simulink library "wtd_library_ver1"  (R2014b)
settings: Solver=ode45  StartTime=0.0  StopTime=10.0  RelTol=1e-3
undefined symbols (not defined in the file or in its folder): clearaugYMatrix, complexPower, dwo, faultaugYMatrix, genTranReactance, invclearaugYMatrix, invfaultaugYMatrix, invsystemaugYMatrix, j, nodeVoltage, noGridNodes, pffault_set_global, s3cc, tho
undefined symbols (not defined in the file): baseSystemPower, internalGenVoltage, pitchAngleVec, systemFrequency, turbSpeedVec, windturbKaParam, windturbKbParam, WTD_Y12, WTD_Y12_2
libraries: simulink x18
(part 3 of 3)

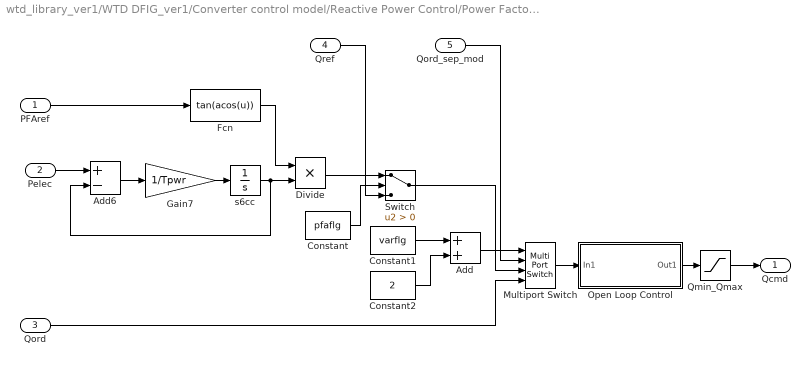
== system wtd_library_ver1/WTD DFIG_ver1/Converter control model/Reactive Power Control/Power Factor Regulator ==
  PFAref : Inport
  Pelec : Inport  Port=2
  Qord : Inport  Port=3
  Qref : Inport  Port=4
  Qord_sep_mod : Inport  Port=5
  Add : Sum
  Add6 : Sum  Inputs=+-
  Constant : Constant  Value=pfaflg
  Constant1 : Constant  Value=varflg
  Constant2 : Constant  Value=2
  Divide : Product  Inputs=**
  Fcn : Fcn  Expr=tan(acos(u))
  Gain7 : Gain  Gain=1/Tpwr
  Multiport Switch : MultiPortSwitch
  Open Loop Control : Subsystem
  Qmin_Qmax : Saturate  UpperLimit=Qmax  LowerLimit=Qmin
  Switch : Switch  Criteria=u2 > Threshold
  s6cc : Integrator  InitialCondition=s6cc
  Qcmd : Outport
  wires:
  Pelec/1 -> Add6/1
  s6cc/1 -> Divide/2, Add6/2
  Add6/1 -> Gain7/1
  Gain7/1 -> s6cc/1
  Qmin_Qmax/1 -> Qcmd/1
  Open Loop Control/1(Out1) -> Qmin_Qmax/1
  Multiport Switch/1 -> Open Loop Control/1(In1)
  Qord/1 -> Multiport Switch/4
  Switch/1 -> Multiport Switch/3
  Qord_sep_mod/1 -> Multiport Switch/2
  Add/1 -> Multiport Switch/1
  Constant2/1 -> Add/2
  Constant1/1 -> Add/1
  Qref/1 -> Switch/3
  Constant/1 -> Switch/2
  Divide/1 -> Switch/1
  Fcn/1 -> Divide/1
  PFAref/1 -> Fcn/1

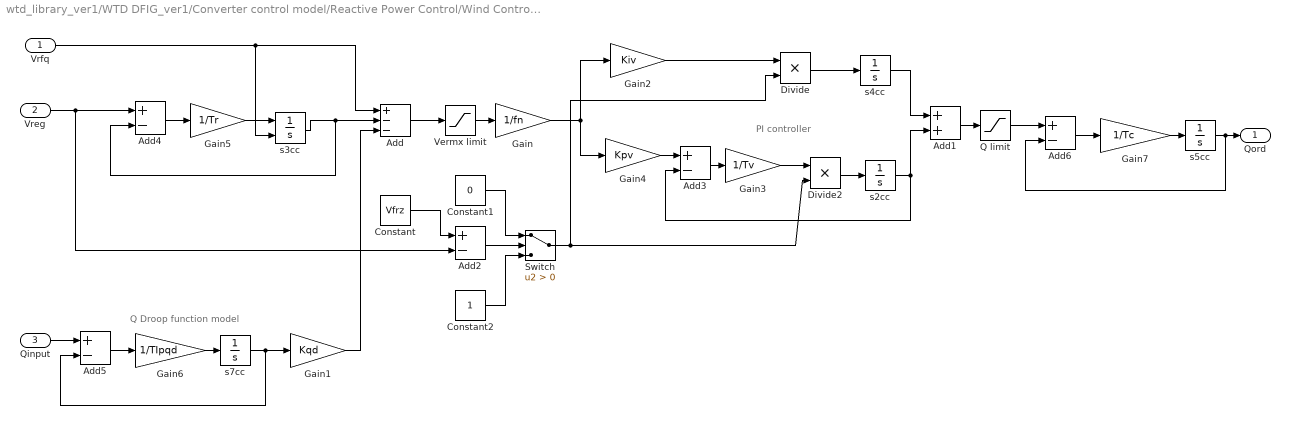
== system wtd_library_ver1/WTD DFIG_ver1/Converter control model/Reactive Power Control/Wind Control Emulator ==
  note: PI controller
  note: Q Droop function model
  Vrfq : Inport
  Vreg : Inport  Port=2
  Qinput : Inport  Port=3
  Add : Sum  Inputs=+--
  Add1 : Sum
  Add{2..6} (5 alike) : Sum  Inputs=+-
  Constant : Constant  Value=Vfrz
  Constant1 : Constant  Value=0
  Constant2 : Constant
  Divide : Product  Inputs=**
  Divide2 : Product  Inputs=**
  Gain : Gain  Gain=1/fn
  Gain1 : Gain  Gain=Kqd
  Gain2 : Gain  Gain=Kiv
  Gain3 : Gain  Gain=1/Tv
  Gain4 : Gain  Gain=Kpv
  Gain5 : Gain  Gain=1/Tr
  Gain6 : Gain  Gain=1/TIpqd
  Gain7 : Gain  Gain=1/Tc
  Q limit : Saturate  UpperLimit=Qmax  LowerLimit=Qmin
  Switch : Switch  Criteria=u2 > Threshold
  Vermx limit : Saturate  UpperLimit=Vermx  LowerLimit=Vermn
  s2cc : Integrator  InitialCondition=s2cc
  s3cc : Integrator  InitialConditionSource=external  InitialCondition=s3cc
  s4cc : Integrator  InitialCondition=s4cc
  s5cc : Integrator  InitialCondition=s5cc
  s7cc : Integrator  InitialCondition=s7cc
  Qord : Outport
  wires:
  Q limit/1 -> Add6/1
  s5cc/1 -> Qord/1, Add6/2
  Add6/1 -> Gain7/1
  Gain7/1 -> s5cc/1
  Qinput/1 -> Add5/1
  s7cc/1 -> Gain1/1, Add5/2
  Add5/1 -> Gain6/1
  Gain6/1 -> s7cc/1
  s3cc/1 -> Add/2, Add4/2
  Add4/1 -> Gain5/1
  Gain5/1 -> s3cc/1
  Divide/1 -> s4cc/1
  Gain2/1 -> Divide/1
  Constant2/1 -> Switch/3
  Switch/1 -> Divide2/2, Divide/2
  Gain4/1 -> Add3/1
  Add3/1 -> Gain3/1
  s2cc/1 -> Add1/2, Add3/2
  Divide2/1 -> s2cc/1
  Gain3/1 -> Divide2/1
  Constant1/1 -> Switch/1
  Constant/1 -> Add2/1
  Add2/1 -> Switch/2
  Add1/1 -> Q limit/1
  s4cc/1 -> Add1/1
  Gain/1 -> Gain2/1, Gain4/1
  Gain1/1 -> Add/3
  Vermx limit/1 -> Gain/1
  Add/1 -> Vermx limit/1
  Vreg/1 -> Add4/1, Add2/2
  Vrfq/1 -> Add/1, s3cc/2

== system wtd_library_ver1/WTD DFIG_ver1/WT_model/Active Power Control Emulator/Subsystem ==
  pavf : Inport
  fbu : Inport  Port=2
  0 : Constant  Value=0
  1 : Constant
  Add : Sum  Inputs=+-
  Divide : Product  Inputs=**
  Fd : Constant  Value=Fd
  Lookup Table1 : Lookup  InputValues=[0.95 Fa Fb Fc Fd]  Table=[Pa Pa Pbc Pbc Pd]
  Switch : Switch  Criteria=u2 > Threshold
  Timer 1 s : Subsystem
  pset : Outport
  f_trip : Outport  Port=2
  wires:
  1/1 -> Switch/1
  0/1 -> Switch/3
  Add/1 -> Switch/2
  Fd/1 -> Add/2
  Switch/1 -> Timer 1 s/1(enable)
  Divide/1 -> pset/1
  Lookup Table1/1 -> Divide/2
  pavf/1 -> Divide/1
  fbu/1 -> Lookup Table1/1, Add/1
  Timer 1 s/1(f_trip) -> f_trip/1

== system wtd_library_ver1/WTD DFIG_ver1/WT_model/Active Power Control Emulator/Wind power model1 ==
  vw : Inport
  Cpmax : Constant  Value=0.5173
  Divide1 : Product  Inputs=***
  Fcn : Fcn  Expr=u^3
  Ka : Constant  Value=Ka(co_node)
  Pmech : Outport
  wires:
  Cpmax/1 -> Divide1/2
  Divide1/1 -> Pmech/1  "Pmech"
  Fcn/1 -> Divide1/1
  Ka/1 -> Divide1/3
  vw/1 -> Fcn/1

== system wtd_library_ver1/WTD DFIG_ver1/WT_model/Pitch compensator/Saturation ==
  z : Inport
  ymax : Inport  Port=2
  ymin : Inport  Port=3
  y : Inport  Port=4
  Add1 : Sum
  Add2 : Sum  Inputs=-+
  Add3 : Sum  Inputs=+-
  Add4 : Sum
  Compare To Zero : simulink/Logic and Bit Operations/Compare To Zero  relop=<  OutDataTypeStr=uint8
  Compare To Zero1 : simulink/Logic and Bit Operations/Compare To Zero  relop=<  OutDataTypeStr=uint8
  Compare To Zero{2..5} (4 alike) : simulink/Logic and Bit Operations/Compare To Zero  relop=>  OutDataTypeStr=uint8
  Product : Product  RndMeth=Zero
  ysw : Outport
  wires:
  Product/1 -> ysw/1
  Compare To Zero5/1 -> Product/2
  Compare To Zero2/1 -> Product/1
  Add4/1 -> Compare To Zero5/1
  Compare To Zero3/1 -> Add4/2
  Compare To Zero4/1 -> Add4/1
  Add3/1 -> Compare To Zero3/1
  ymin/1 -> Add3/2
  Add1/1 -> Compare To Zero2/1
  Compare To Zero/1 -> Add1/2
  Compare To Zero1/1 -> Add1/1
  z/1 -> Compare To Zero4/1, Compare To Zero/1
  Add2/1 -> Compare To Zero1/1
  ymax/1 -> Add2/1
  y/1 -> Add3/1, Add2/2

== system wtd_library_ver1/WTD DFIG_ver1/WT_model/Pitch controller/Saturation ==
  z : Inport
  ymax : Inport  Port=2
  ymin : Inport  Port=3
  y : Inport  Port=4
  Add1 : Sum
  Add2 : Sum  Inputs=-+
  Add3 : Sum  Inputs=+-
  Add4 : Sum
  Compare To Zero : simulink/Logic and Bit Operations/Compare To Zero  relop=<  OutDataTypeStr=uint8
  Compare To Zero1 : simulink/Logic and Bit Operations/Compare To Zero  relop=<  OutDataTypeStr=uint8
  Compare To Zero{2..5} (4 alike) : simulink/Logic and Bit Operations/Compare To Zero  relop=>  OutDataTypeStr=uint8
  Product : Product  RndMeth=Zero
  ysw : Outport
  wires:
  Product/1 -> ysw/1
  Compare To Zero5/1 -> Product/2
  Compare To Zero2/1 -> Product/1
  Add4/1 -> Compare To Zero5/1
  Compare To Zero3/1 -> Add4/2
  Compare To Zero4/1 -> Add4/1
  Add3/1 -> Compare To Zero3/1
  ymin/1 -> Add3/2
  Add1/1 -> Compare To Zero2/1
  Compare To Zero/1 -> Add1/2
  Compare To Zero1/1 -> Add1/1
  z/1 -> Compare To Zero4/1, Compare To Zero/1
  Add2/1 -> Compare To Zero1/1
  ymax/1 -> Add2/1
  y/1 -> Add3/1, Add2/2

== system wtd_library_ver1/WTD DFIG_ver1/WT_model/Torque controller/Saturation ==
  z : Inport
  ymax : Inport  Port=2
  ymin : Inport  Port=3
  y : Inport  Port=4
  Add1 : Sum
  Add2 : Sum  Inputs=-+
  Add3 : Sum  Inputs=+-
  Add4 : Sum
  Compare To Zero : simulink/Logic and Bit Operations/Compare To Zero  relop=<  OutDataTypeStr=uint8
  Compare To Zero1 : simulink/Logic and Bit Operations/Compare To Zero  relop=<  OutDataTypeStr=uint8
  Compare To Zero{2..5} (4 alike) : simulink/Logic and Bit Operations/Compare To Zero  relop=>  OutDataTypeStr=uint8
  Product : Product  RndMeth=Zero
  ysw : Outport
  wires:
  Product/1 -> ysw/1
  Compare To Zero5/1 -> Product/2
  Compare To Zero2/1 -> Product/1
  Add4/1 -> Compare To Zero5/1
  Compare To Zero3/1 -> Add4/2
  Compare To Zero4/1 -> Add4/1
  Add3/1 -> Compare To Zero3/1
  ymin/1 -> Add3/2
  Add1/1 -> Compare To Zero2/1
  Compare To Zero/1 -> Add1/2
  Compare To Zero1/1 -> Add1/1
  z/1 -> Compare To Zero4/1, Compare To Zero/1
  Add2/1 -> Compare To Zero1/1
  ymax/1 -> Add2/1
  y/1 -> Add3/1, Add2/2

== system wtd_library_ver1/WTD DFIG_ver1/WT_model/Wind power model/Cp & lambda ==
  theta : Inport
  vw : Inport  Port=2
  w : Inport  Port=3
  Product : Product  Inputs=3  Multiplication=Matrix(*)  RndMeth=Zero
  Vektor lambda : Subsystem
  Vektor theta : Subsystem
  cp_koeficijenti : Constant  Value=alpha
  Cp : Outport
  lambda : Outport  Port=2
  wires:
  Vektor lambda/1(lambda) -> lambda/1
  Product/1 -> Cp/1
  w/1 -> Vektor lambda/2(w)
  vw/1 -> Vektor lambda/1(vw)
  theta/1 -> Vektor theta/1(theta)
  cp_koeficijenti/1 -> Product/2
  Vektor lambda/2(lambda_na_j) -> Product/3
  Vektor theta/1(theta_na_i) -> Product/1

== system wtd_library_ver1/WTD DFIG_ver1/Converter control model/Reactive Power Control/Power Factor Regulator/Open Loop Control ==
  In1 : Inport
  Out1 : Outport
  wires:
  In1/1 -> Out1/1

== system wtd_library_ver1/WTD DFIG_ver1/WT_model/Active Power Control Emulator/Subsystem/Timer 1 s ==
  enable : Inport
  Add : Sum  Inputs=-+
  Constant2 : Constant
  Constant3 : Constant  Value=0
  Enabled Subsystem : Subsystem  TreatAsAtomicUnit=on
  Enabled Subsystem1 : Subsystem  TreatAsAtomicUnit=on
  Hit Crossing : HitCross  HitCrossingDirection=rising
  Switch : Switch  Threshold=1
  f_trip : Outport
  wires:
  Hit Crossing/1 -> Enabled Subsystem/Enable
  Enabled Subsystem/1(timer) -> Add/1
  Enabled Subsystem1/1(timer) -> Add/2
  Switch/1 -> f_trip/1
  Add/1 -> Switch/2
  Constant2/1 -> Switch/1
  Constant3/1 -> Switch/3
  enable/1 -> Hit Crossing/1, Enabled Subsystem1/Enable

== system wtd_library_ver1/WTD DFIG_ver1/WT_model/Wind power model/Cp & lambda/Vektor lambda ==
  vw : Inport
  w : Inport  Port=2
  Constant1 : Constant
  Divide1 : Product  Inputs=/*
  Divide2 : Product  Inputs=**
  Divide3 : Product  Inputs=**
  Divide4 : Product  Inputs=**
  Gain : Gain  Gain=Kb(co_node)
  Reshape : Reshape  OutputDimensionality=Customize  OutputDimensions=[5,1]
  Vector Concatenate : Concatenate  NumInputs=5
  lambda : Outport
  lambda_na_j : Outport  Port=2
  wires:
  Reshape/1 -> lambda_na_j/1
  Vector Concatenate/1 -> Reshape/1
  vw/1 -> Divide1/1
  w/1 -> Divide1/2
  Divide4/1 -> Vector Concatenate/5
  Divide3/1 -> Divide4/1, Vector Concatenate/4
  Divide2/1 -> Divide3/1, Vector Concatenate/3
  Gain/1 -> lambda/1, Divide4/2, Divide3/2, Divide2/2, Divide2/1, Vector Concatenate/2
  Constant1/1 -> Vector Concatenate/1
  Divide1/1 -> Gain/1

== system wtd_library_ver1/WTD DFIG_ver1/WT_model/Wind power model/Cp & lambda/Vektor theta ==
  theta : Inport
  Constant1 : Constant
  Divide2 : Product  Inputs=**
  Divide3 : Product  Inputs=**
  Divide4 : Product  Inputs=**
  Reshape : Reshape  OutputDimensionality=Customize  OutputDimensions=[1,5]
  Vector Concatenate : Concatenate  NumInputs=5
  theta_na_i : Outport
  wires:
  Reshape/1 -> theta_na_i/1
  Vector Concatenate/1 -> Reshape/1
  Constant1/1 -> Vector Concatenate/1
  Divide2/1 -> Vector Concatenate/3, Divide3/1
  Divide3/1 -> Vector Concatenate/4, Divide4/1
  Divide4/1 -> Vector Concatenate/5
  theta/1 -> Vector Concatenate/2, Divide2/1, Divide2/2, Divide3/2, Divide4/2

== system wtd_library_ver1/WTD DFIG_ver1/WT_model/Active Power Control Emulator/Subsystem/Timer 1 s/Enabled Subsystem ==
  Enable : EnablePort
  Constant : Constant
  Enabled Subsystem : Subsystem  TreatAsAtomicUnit=on
  timer : Outport
  wires:
  Enabled Subsystem/1(Out1) -> timer/1
  Constant/1 -> Enabled Subsystem/Enable

== system wtd_library_ver1/WTD DFIG_ver1/WT_model/Active Power Control Emulator/Subsystem/Timer 1 s/Enabled Subsystem1 ==
  Enable : EnablePort
  Clock : Clock
  timer : Outport
  wires:
  Clock/1 -> timer/1

== system wtd_library_ver1/WTD DFIG_ver1/WT_model/Active Power Control Emulator/Subsystem/Timer 1 s/Enabled Subsystem/Enabled Subsystem ==
  Enable : EnablePort
  Clock : Clock
  Out1 : Outport
  wires:
  Clock/1 -> Out1/1
